simulink subsystem "MC_OFF"  (R2023b)
settings: Solver=VariableStepAuto  StartTime=0.0  StopTime=10.0  RelTol=1e-3
settings Model: Creator=nickj  LastModifiedBy=heyka

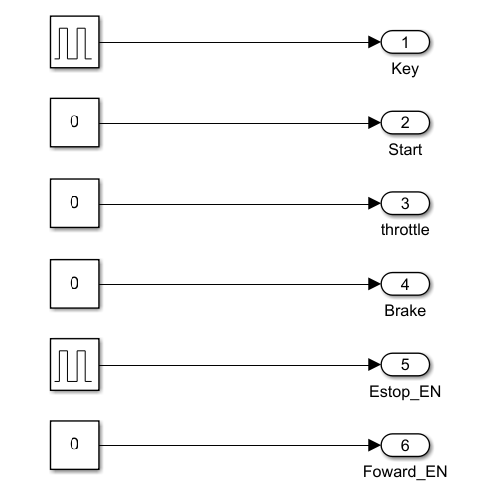
[thumbnail: Simulink's stored preview of the top-level diagram]
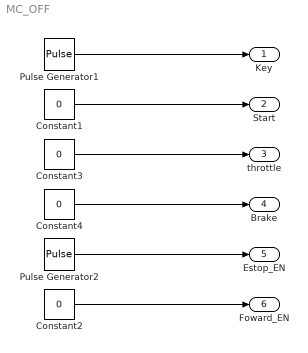
== system MC_OFF ==
  Constant{1..4} (4 alike) : Constant  Value=0
  Pulse Generator1 : DiscretePulseGenerator  PulseType=Time based  Period=8  PulseWidth=25  PhaseDelay=4
  Pulse Generator2 : DiscretePulseGenerator  PulseType=Time based  Period=4  PulseWidth=50
  Key : Outport
  Start : Outport  Port=2
  throttle : Outport  Port=3
  Brake : Outport  Port=4
  Estop_EN : Outport  Port=5
  Foward_EN : Outport  Port=6
  wires:
  Constant4/1 -> Brake/1
  Constant3/1 -> throttle/1
  Constant2/1 -> Foward_EN/1
  Constant1/1 -> Start/1
  Pulse Generator2/1 -> Estop_EN/1
  Pulse Generator1/1 -> Key/1
